simulink model "simulink_template"  (R2021a)
settings: Solver=ode4  StartTime=0.0  StopTime=2  FixedStep=.01  RelTol=1e-3
settings Model: Creator=Cameron  LastModifiedBy=elissaito
settings SolverCC: AlgebraicLoopSolver=TrustRegion
settings DataIOCC: ReturnWorkspaceOutputs=off
settings DebuggingCC: SFMachineParentedDataDiag=warning  ArithmeticOperatorsInVariantConditions=warning
settings SFSimCC: SimUseLocalCustomCode=off  CustomCodeUndefinedFunction=UseInterfaceOnly
settings RTWCC: RTWUseLocalCustomCode=off
settings CodeAppCC: StateflowObjectComments=on

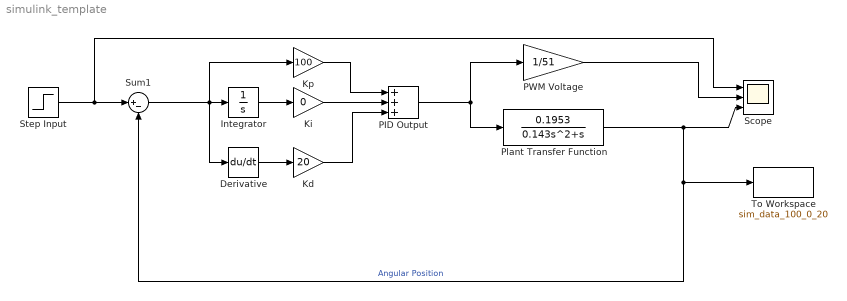
== system simulink_template ==
  Derivative : Derivative
  Integrator : Integrator
  Kd : Gain  Gain=20
  Ki : Gain  Gain=0
  Kp : Gain  Gain=100
  PID Output : Sum  Inputs=+++
  PWM Voltage : Gain  Gain=1/51
  Plant Transfer Function : TransferFcn  Numerator=[0.1953]  Denominator=[0.143 1 0]
  Scope : Scope  NumInputPorts=3
  Step Input : Step  Time=0  After=pi/2  SampleTime=0
  Sum1 : Sum  Inputs=|+-
  To Workspace : ToWorkspace  VariableName=sim_data_100_0_20  SaveFormat=Timeseries  SampleTime=-1
  wires:
  Step Input/1 -> Scope/1, Sum1/1
  Plant Transfer Function/1 -> Scope/3, To Workspace/1, Sum1/2  "Angular Position"
  PWM Voltage/1 -> Scope/2
  Ki/1 -> PID Output/2
  Kp/1 -> PID Output/1
  Sum1/1 -> Integrator/1, Derivative/1, Kp/1
  Integrator/1 -> Ki/1
  Derivative/1 -> Kd/1
  Kd/1 -> PID Output/3
  PID Output/1 -> Plant Transfer Function/1, PWM Voltage/1
